simulink model "point_mass_EOM"  (R2019b)
settings: Solver=VariableStepAuto  StartTime=0.0  StopTime=10.0  RelTol=1e-3  EnableMultiTasking=on
undefined symbols (not defined in the file): alpha_T, CD_0, chi_init, CL_0, CL_alpha, g, gamma_init, h_init, k, m, T_0, T_deltaT, V_init
libraries: aerolibatmos2 x1
settings Model: Creator=Christoph Göttlicher  LastModifiedBy=YUMU
settings DataIOCC: LimitDataPoints=on  ReturnWorkspaceOutputs=off
settings OptimizationCC: LifeSpan=inf
settings DebuggingCC: AllowSymbolicDim=off  SFUnexpectedBacktrackingDiag=warning  SFNoUnconditionalDefaultTransitionDiag=warning  SFExecutionAtInitializationDiag=none  ArithmeticOperatorsInVariantConditions=warning
settings ModelReferenceCC: PropagateSignalLabelsOutOfModel=off
settings SFSimCC: SimUseLocalCustomCode=off  CustomCodeUndefinedFunction=UseInterfaceOnly
settings RTWCC: RTWUseLocalCustomCode=off
settings CodeAppCC: StateflowObjectComments=on
settings GRTTargetCC: TargetLangStandard=C89/C90 (ANSI)
settings ConfigComp: CovMetricSettings=dw  CovHtmlReporting=on  CovSaveCumulativeToWorkspaceVar=on  CovSaveSingleToWorkspaceVar=on  CovExternalEMLEnable=off

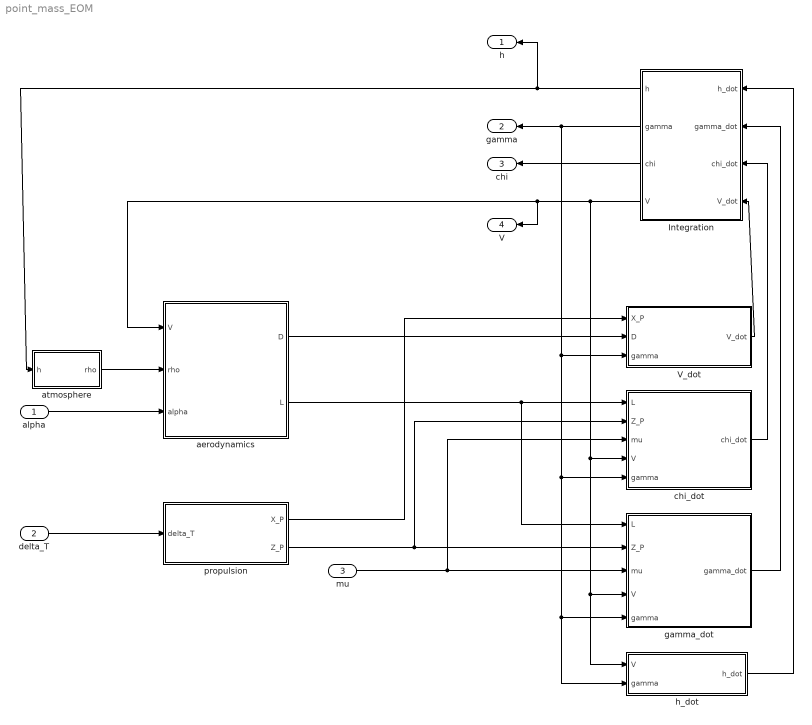
== system point_mass_EOM ==
  alpha : Inport
  delta_T : Inport  Port=2
  mu : Inport  Port=3
  Integration : Subsystem
  V_dot : Subsystem
  aerodynamics : Subsystem
  atmosphere : Subsystem
  chi_dot : Subsystem
  gamma_dot : Subsystem
  h_dot : Subsystem
  propulsion : Subsystem
  h : Outport
  gamma : Outport  Port=2
  chi : Outport  Port=3
  V : Outport  Port=4
  wires:
  alpha/1 -> aerodynamics/3(alpha)
  delta_T/1 -> propulsion/1(delta_T)
  V_dot/1(V_dot) -> Integration/4(V_dot)
  chi_dot/1(chi_dot) -> Integration/3(chi_dot)
  gamma_dot/1(gamma_dot) -> Integration/2(gamma_dot)
  h_dot/1(h_dot) -> Integration/1(h_dot)
  Integration/4(V) -> V/1, aerodynamics/1(V), chi_dot/4(V), gamma_dot/4(V), h_dot/1(V)
  Integration/3(chi) -> chi/1
  Integration/1(h) -> atmosphere/1(h), h/1
  Integration/2(gamma) -> chi_dot/5(gamma), gamma_dot/5(gamma), h_dot/2(gamma), V_dot/3(gamma), gamma/1
  aerodynamics/2(L) -> gamma_dot/1(L), chi_dot/1(L)
  aerodynamics/1(D) -> V_dot/2(D)
  propulsion/1(X_P) -> V_dot/1(X_P)
  propulsion/2(Z_P) -> chi_dot/2(Z_P), gamma_dot/2(Z_P)
  mu/1 -> chi_dot/3(mu), gamma_dot/3(mu)
  atmosphere/1(rho) -> aerodynamics/2(rho)

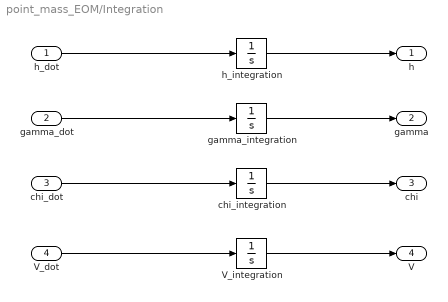
== system point_mass_EOM/Integration ==
  h_dot : Inport
  gamma_dot : Inport  Port=2
  chi_dot : Inport  Port=3
  V_dot : Inport  Port=4
  V_integration : Integrator  InitialCondition=V_init  ContinuousStateAttributes='V'
  chi_integration : Integrator  InitialCondition=chi_init  ContinuousStateAttributes='chi'
  gamma_integration : Integrator  InitialCondition=gamma_init  ContinuousStateAttributes='gamma'
  h_integration : Integrator  InitialCondition=h_init  ContinuousStateAttributes='h'
  h : Outport
  gamma : Outport  Port=2
  chi : Outport  Port=3
  V : Outport  Port=4
  wires:
  V_dot/1 -> V_integration/1
  V_integration/1 -> V/1
  h_integration/1 -> h/1
  h_dot/1 -> h_integration/1
  gamma_dot/1 -> gamma_integration/1
  gamma_integration/1 -> gamma/1
  chi_integration/1 -> chi/1
  chi_dot/1 -> chi_integration/1

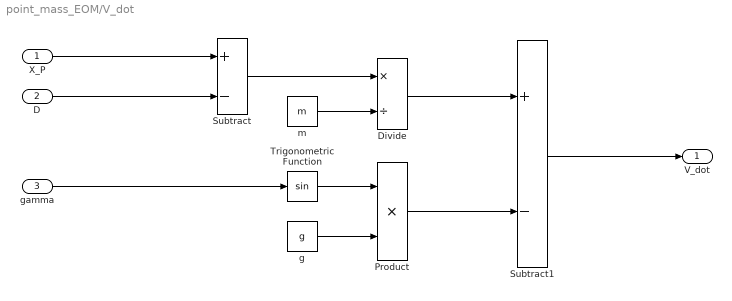
== system point_mass_EOM/V_dot ==
  X_P : Inport
  D : Inport  Port=2
  gamma : Inport  Port=3
  Divide : Product  Inputs=*/
  Product : Product
  Subtract : Sum  Inputs=+-
  Subtract1 : Sum  Inputs=+-
  Trigonometric Function : Trigonometry
  g : Constant  Value=g
  m : Constant  Value=m
  V_dot : Outport
  wires:
  X_P/1 -> Subtract/1
  D/1 -> Subtract/2
  Subtract/1 -> Divide/1
  m/1 -> Divide/2
  Divide/1 -> Subtract1/1
  gamma/1 -> Trigonometric Function/1
  Trigonometric Function/1 -> Product/1
  g/1 -> Product/2
  Product/1 -> Subtract1/2
  Subtract1/1 -> V_dot/1

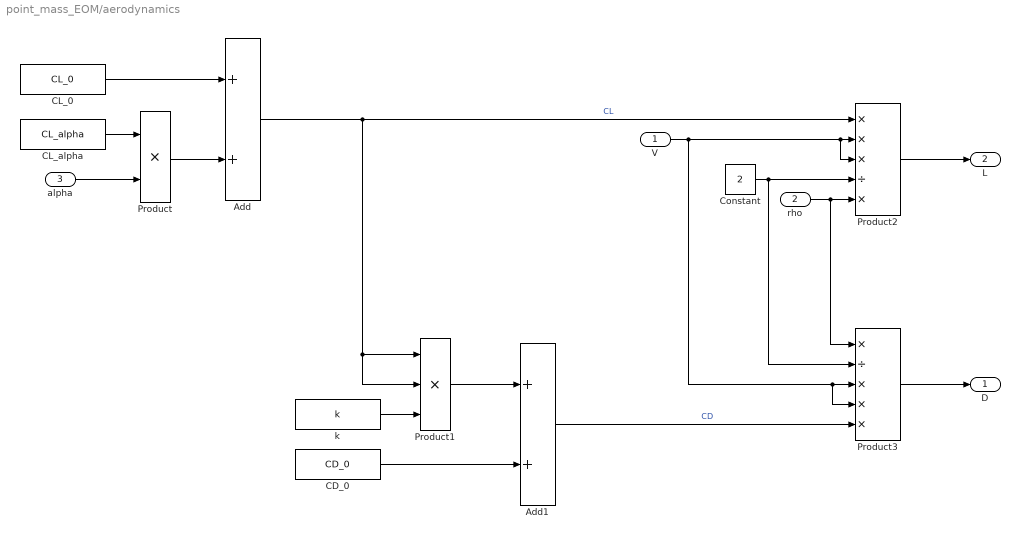
== system point_mass_EOM/aerodynamics ==
  V : Inport
  rho : Inport  Port=2
  alpha : Inport  Port=3
  Add : Sum
  Add1 : Sum
  CD_0 : Constant  Value=CD_0
  CL_0 : Constant  Value=CL_0
  CL_alpha : Constant  Value=CL_alpha
  Constant : Constant  Value=2
  Product : Product
  Product1 : Product  Inputs=3
  Product2 : Product  Inputs=***/*
  Product3 : Product  Inputs=*/***
  k : Constant  Value=k
  D : Outport
  L : Outport  Port=2
  wires:
  alpha/1 -> Product/2
  CL_alpha/1 -> Product/1
  Product/1 -> Add/2
  CL_0/1 -> Add/1
  Add/1 -> Product2/1, Product1/1, Product1/2  "CL"
  CD_0/1 -> Add1/2
  Product1/1 -> Add1/1
  k/1 -> Product1/3
  rho/1 -> Product3/1, Product2/5
  Constant/1 -> Product3/2, Product2/4
  Product2/1 -> L/1
  V/1 -> Product3/4, Product3/3, Product2/3, Product2/2
  Product3/1 -> D/1
  Add1/1 -> Product3/5  "CD"

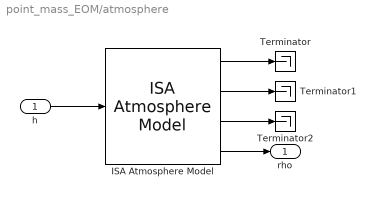
== system point_mass_EOM/atmosphere ==
  h : Inport
  ISA Atmosphere Model : aerolibatmos2/ISA Atmosphere Model  custom=off  g=9.80665  gamma=1.4  R=287.0531  L=0.0065  h_trop=11000  h_strat=20000  rho0=1.225  P0=101325  T0=288.15  h0=0
      settings: SourceProductName=Aerospace Blockset
  Terminator : Terminator
  Terminator1 : Terminator
  Terminator2 : Terminator
  rho : Outport
  wires:
  ISA Atmosphere Model/4 -> rho/1
  ISA Atmosphere Model/2 -> Terminator1/1
  ISA Atmosphere Model/1 -> Terminator/1
  ISA Atmosphere Model/3 -> Terminator2/1
  h/1 -> ISA Atmosphere Model/1

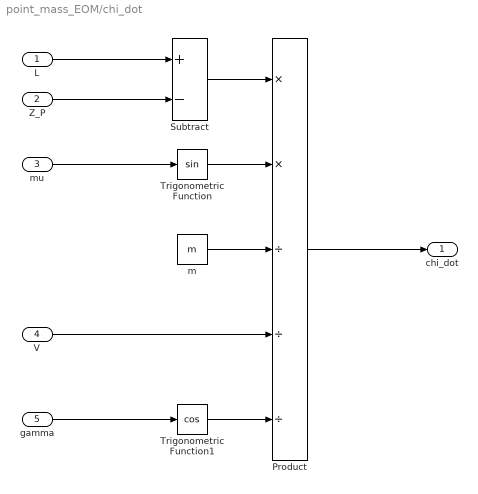
== system point_mass_EOM/chi_dot ==
  L : Inport
  Z_P : Inport  Port=2
  mu : Inport  Port=3
  V : Inport  Port=4
  gamma : Inport  Port=5
  Product : Product  Inputs=**///
  Subtract : Sum  Inputs=+-
  Trigonometric Function : Trigonometry
  Trigonometric Function1 : Trigonometry  Operator=cos
  m : Constant  Value=m
  chi_dot : Outport
  wires:
  L/1 -> Subtract/1
  Z_P/1 -> Subtract/2
  mu/1 -> Trigonometric Function/1
  Trigonometric Function/1 -> Product/2
  Subtract/1 -> Product/1
  m/1 -> Product/3
  gamma/1 -> Trigonometric Function1/1
  V/1 -> Product/4
  Trigonometric Function1/1 -> Product/5
  Product/1 -> chi_dot/1

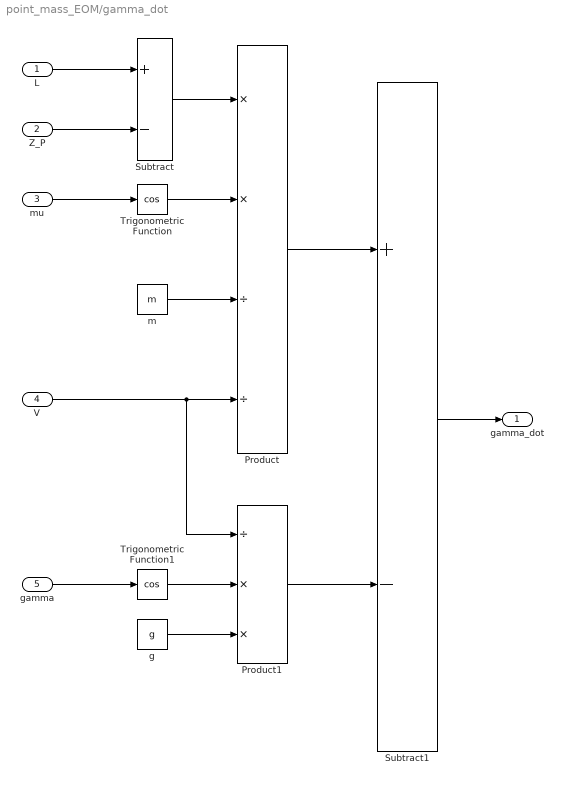
== system point_mass_EOM/gamma_dot ==
  L : Inport
  Z_P : Inport  Port=2
  mu : Inport  Port=3
  V : Inport  Port=4
  gamma : Inport  Port=5
  Product : Product  Inputs=**//
  Product1 : Product  Inputs=/**
  Subtract : Sum  Inputs=+-
  Subtract1 : Sum  Inputs=+-
  Trigonometric Function : Trigonometry  Operator=cos
  Trigonometric Function1 : Trigonometry  Operator=cos
  g : Constant  Value=g
  m : Constant  Value=m
  gamma_dot : Outport
  wires:
  L/1 -> Subtract/1
  Z_P/1 -> Subtract/2
  mu/1 -> Trigonometric Function/1
  Subtract/1 -> Product/1
  Trigonometric Function/1 -> Product/2
  V/1 -> Product1/1, Product/4
  m/1 -> Product/3
  Product/1 -> Subtract1/1
  Trigonometric Function1/1 -> Product1/2
  gamma/1 -> Trigonometric Function1/1
  g/1 -> Product1/3
  Product1/1 -> Subtract1/2
  Subtract1/1 -> gamma_dot/1

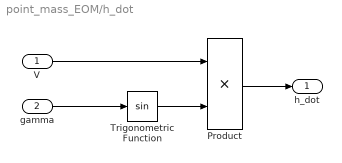
== system point_mass_EOM/h_dot ==
  V : Inport
  gamma : Inport  Port=2
  Product : Product
  Trigonometric Function : Trigonometry
  h_dot : Outport
  wires:
  gamma/1 -> Trigonometric Function/1
  Trigonometric Function/1 -> Product/2
  Product/1 -> h_dot/1
  V/1 -> Product/1

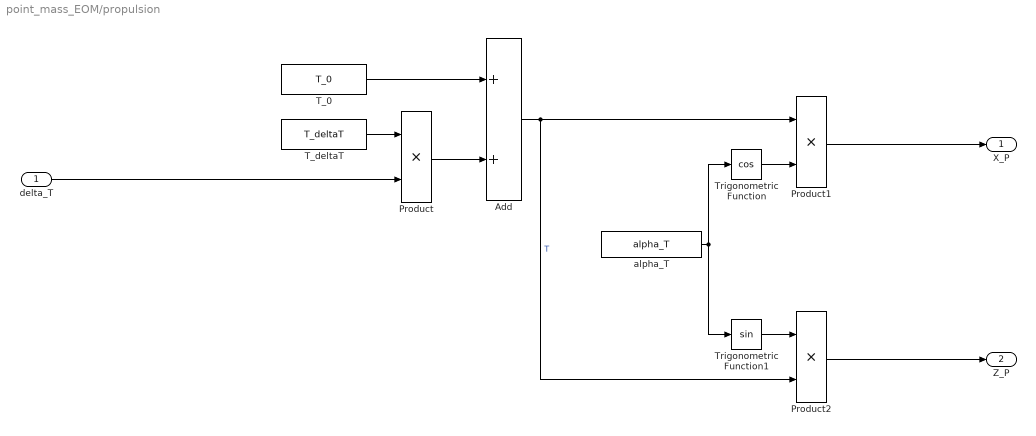
== system point_mass_EOM/propulsion ==
  delta_T : Inport
  Add : Sum
  Product : Product
  Product1 : Product
  Product2 : Product
  T_0 : Constant  Value=T_0
  T_deltaT : Constant  Value=T_deltaT
  Trigonometric Function : Trigonometry  Operator=cos
  Trigonometric Function1 : Trigonometry
  alpha_T : Constant  Value=alpha_T
  X_P : Outport
  Z_P : Outport  Port=2
  wires:
  Add/1 -> Product2/2, Product1/1  "T"
  T_0/1 -> Add/1
  Product/1 -> Add/2
  T_deltaT/1 -> Product/1
  delta_T/1 -> Product/2
  Product1/1 -> X_P/1
  Trigonometric Function/1 -> Product1/2
  alpha_T/1 -> Trigonometric Function1/1, Trigonometric Function/1
  Trigonometric Function1/1 -> Product2/1
  Product2/1 -> Z_P/1
